simulink model "golayCorrelator"  (R2014b)
settings: Solver=FixedStepDiscrete  StartTime=0  StopTime=10000  RelTol=1e-3
values from neighbouring files (symbols this model uses):
  D_128 = [ 1,  8,  2,  4, 16, 32, 64]    [golay.m]    (also in rev0BB_setup.m; rev0BB_startup.m = D_128 .* 4)
  W_128 = [-1, -1, -1, -1, +1, -1, -1]    [golay.m]    (also in rev0BB_setup.m; rev0BB_startup.m)
libraries: golayLib x7, commdigbbndpm3 x2, dspsigops x2, commchan3 x1, dspmlti4 x1, commrflib2 x1
settings Model: Creator=cyarp  LastModifiedBy=cyarp

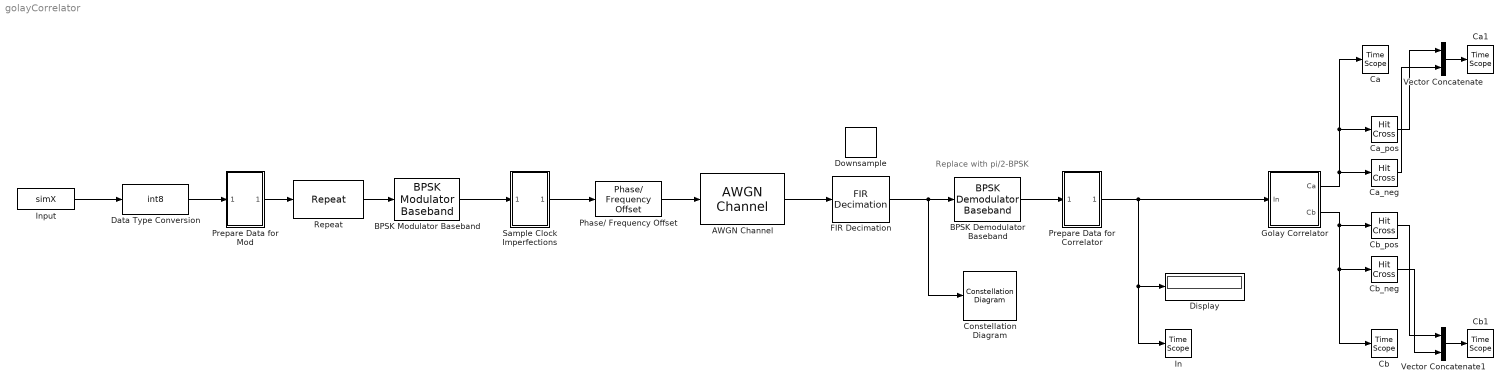
== system golayCorrelator ==
  note: Replace with pi/2-BPSK
  AWGN Channel : commchan3/AWGN Channel  InputProcessing=Columns as channels (frame based)  seed=67  noiseMode="Signal to noise ratio  (Eb/No)"  EbNodB=0  EsNodB=10  SNRdB=10  bitsPerSym=1  Ps=1  Tsym=1  variance=1
  BPSK Demodulator Baseband : commdigbbndpm3/BPSK Demodulator Baseband  Ph=0  DecType=Hard decision  VarSource=Dialog  Variance=1  outDtype=Inherit via internal rule  derotateFactorWordLen=16
  BPSK Modulator Baseband : commdigbbndpm3/BPSK Modulator Baseband  Ph=0  outDtype=double  outWordLen=16  outUDDataType=sfix(16)  outFracLenMode=Best precision  outFracLen=15
  Ca : TimeScope  DefaultConfigurationName=spbscopes.TimeScopeBlockCfg
  Ca1 : TimeScope  DefaultConfigurationName=spbscopes.TimeScopeBlockCfg
  Ca_neg : HitCross  HitCrossingOffset=-50  HitCrossingDirection=falling
  Ca_pos : HitCross  HitCrossingOffset=50  HitCrossingDirection=rising
  Cb : TimeScope  DefaultConfigurationName=spbscopes.TimeScopeBlockCfg
  Cb1 : TimeScope  DefaultConfigurationName=spbscopes.TimeScopeBlockCfg
  Cb_neg : HitCross  HitCrossingOffset=-50  HitCrossingDirection=falling
  Cb_pos : HitCross  HitCrossingOffset=50  HitCrossingDirection=rising
  Constellation Diagram : ConstellationDiagram
  Data Type Conversion : DataTypeConversion  OutDataTypeStr=int8  RndMeth=Nearest
  Display : Display
  Downsample : dspsigops/Downsample  N=4  phase=0  InputProcessing=Columns as channels (frame based)  RateOptions=Allow multirate processing  smode=Allow multirate  fmode=Maintain input frame size  ic=0
  FIR Decimation : dspmlti4/FIR Decimation  h=fir1(45, 0.18)  D=4  filtStruct=Direct form  framing=Allow multirate processing  inputOffset=0  outputBufInitCond=0  InputProcessing=Columns as channels (frame based)  firstCoeffDataTypeStr=Inherit: Same word length as input  firstCoeffLastDataTypeStr=Inherit: Same word length as input  firstCoeffMin=[]  firstCoeffMax=[]  outputDataTypeStr=Inherit: Same as accumulator  outputLastDataTypeStr=Inherit: Same as accumulator  outputMin=[]  outputMax=[]  roundingMode=Floor  overflowMode=off  FilterSource=Specify via dialog  FilterObject=Hm_firdecim
      settings: allowOverrides=off
  Golay Correlator : Subsystem
  In : TimeScope  DefaultConfigurationName=spbscopes.TimeScopeBlockCfg
  Input : FromWorkspace  VariableName=simX  SampleTime=1  Interpolate=off  OutputAfterFinalValue=Holding final value
  Phase/ Frequency Offset : commrflib2/Phase// Frequency Offset  phaseOffset=0  freqPort=off  freqOffset=0
  Prepare Data for Correlator : Subsystem
  Prepare Data for Mod : Subsystem
  Repeat : dspsigops/Repeat  N=4  InputProcessing=Columns as channels (frame based)  RateOptions=Allow multirate processing  ic=0  mode=Unused parameter value
  Sample Clock Imperfections : Subsystem
  Vector Concatenate : Concatenate  Mode=Multidimensional array  ConcatenateDimension=2
  Vector Concatenate1 : Concatenate  Mode=Multidimensional array  ConcatenateDimension=2
  wires:
  Phase/ Frequency Offset/1 -> AWGN Channel/1
  Golay Correlator/1(Ca) -> Ca_neg/1, Ca_pos/1, Ca/1
  Golay Correlator/2(Cb) -> Cb_pos/1, Cb_neg/1, Cb/1
  Input/1 -> Data Type Conversion/1
  AWGN Channel/1 -> FIR Decimation/1
  Data Type Conversion/1 -> Prepare Data for Mod/1(In1)
  Prepare Data for Mod/1(Out1) -> Repeat/1
  BPSK Demodulator Baseband/1 -> Prepare Data for Correlator/1(In1)
  Repeat/1 -> BPSK Modulator Baseband/1
  BPSK Modulator Baseband/1 -> Sample Clock Imperfections/1(In1)
  Sample Clock Imperfections/1(Out1) -> Phase/ Frequency Offset/1
  Prepare Data for Correlator/1(Out1) -> In/1, Display/1, Golay Correlator/1(In)
  FIR Decimation/1 -> Constellation Diagram/1, BPSK Demodulator Baseband/1
  Ca_neg/1 -> Vector Concatenate/2
  Ca_pos/1 -> Vector Concatenate/1
  Vector Concatenate/1 -> Ca1/1
  Cb_pos/1 -> Vector Concatenate1/1
  Cb_neg/1 -> Vector Concatenate1/2
  Vector Concatenate1/1 -> Cb1/1

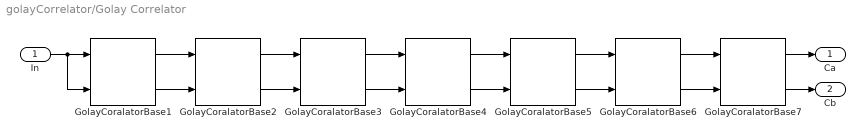
== system golayCorrelator/Golay Correlator ==
  In : Inport
  GolayCoralatorBase1 : golayLib/GolayCoralatorBase  dSub=D_128(1)  wSub=W_128(1)
  GolayCoralatorBase2 : golayLib/GolayCoralatorBase  dSub=D_128(2)  wSub=W_128(2)
  GolayCoralatorBase3 : golayLib/GolayCoralatorBase  dSub=D_128(3)  wSub=W_128(3)
  GolayCoralatorBase4 : golayLib/GolayCoralatorBase  dSub=D_128(4)  wSub=W_128(4)
  GolayCoralatorBase5 : golayLib/GolayCoralatorBase  dSub=D_128(5)  wSub=W_128(5)
  GolayCoralatorBase6 : golayLib/GolayCoralatorBase  dSub=D_128(6)  wSub=W_128(6)
  GolayCoralatorBase7 : golayLib/GolayCoralatorBase  dSub=D_128(7)  wSub=W_128(7)
  Ca : Outport
  Cb : Outport  Port=2
  wires:
  GolayCoralatorBase1/1 -> GolayCoralatorBase2/1
  GolayCoralatorBase1/2 -> GolayCoralatorBase2/2
  GolayCoralatorBase2/1 -> GolayCoralatorBase3/1
  GolayCoralatorBase2/2 -> GolayCoralatorBase3/2
  GolayCoralatorBase5/1 -> GolayCoralatorBase6/1
  GolayCoralatorBase3/1 -> GolayCoralatorBase4/1
  GolayCoralatorBase3/2 -> GolayCoralatorBase4/2
  GolayCoralatorBase4/1 -> GolayCoralatorBase5/1
  GolayCoralatorBase4/2 -> GolayCoralatorBase5/2
  GolayCoralatorBase5/2 -> GolayCoralatorBase6/2
  GolayCoralatorBase6/2 -> GolayCoralatorBase7/2
  GolayCoralatorBase6/1 -> GolayCoralatorBase7/1
  GolayCoralatorBase7/2 -> Cb/1
  GolayCoralatorBase7/1 -> Ca/1
  In/1 -> GolayCoralatorBase1/2, GolayCoralatorBase1/1

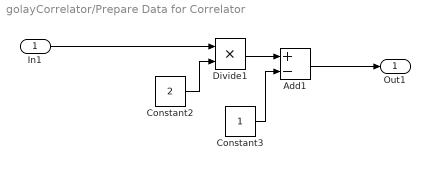
== system golayCorrelator/Prepare Data for Correlator ==
  In1 : Inport
  Add1 : Sum  Inputs=+-
  Constant2 : Constant  Value=2
  Constant3 : Constant
  Divide1 : Product  Inputs=**
  Out1 : Outport
  wires:
  Constant2/1 -> Divide1/2
  Constant3/1 -> Add1/2
  In1/1 -> Divide1/1
  Divide1/1 -> Add1/1
  Add1/1 -> Out1/1

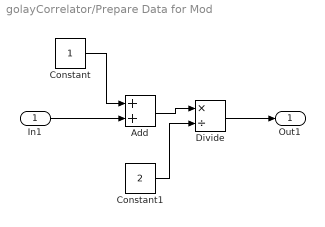
== system golayCorrelator/Prepare Data for Mod ==
  In1 : Inport
  Add : Sum
  Constant : Constant
  Constant1 : Constant  Value=2
  Divide : Product  Inputs=*/
  Out1 : Outport
  wires:
  In1/1 -> Add/2
  Constant/1 -> Add/1
  Add/1 -> Divide/1
  Constant1/1 -> Divide/2
  Divide/1 -> Out1/1

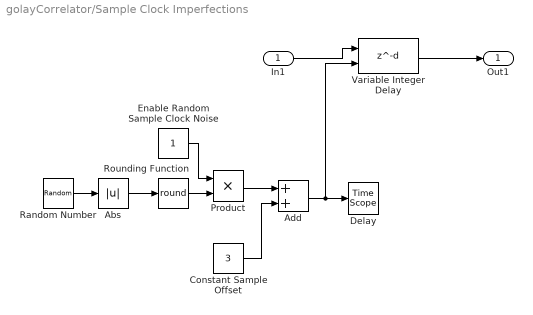
== system golayCorrelator/Sample Clock Imperfections ==
  In1 : Inport
  Abs : Abs
  Add : Sum
  Constant Sample Offset : Constant  Value=3
  Delay : TimeScope  DefaultConfigurationName=spbscopes.TimeScopeBlockCfg
  Enable Random Sample Clock Noise : Constant
  Product : Product
  Random Number : RandomNumber  Mean=1  SampleTime=0.25
  Rounding Function : Rounding  Operator=round
  Variable Integer Delay : Delay  DelayLengthSource=Input port
      settings: InputPortMap=u0,p1
  Out1 : Outport
  wires:
  Abs/1 -> Rounding Function/1
  In1/1 -> Variable Integer Delay/1
  Random Number/1 -> Abs/1
  Variable Integer Delay/1 -> Out1/1
  Add/1 -> Delay/1, Variable Integer Delay/2
  Enable Random Sample Clock Noise/1 -> Product/1
  Constant Sample Offset/1 -> Add/2
  Rounding Function/1 -> Product/2
  Product/1 -> Add/1
